simulink model "first_order_system_parabolicC"  (R2022b)
settings: Solver=VariableStepAuto  StartTime=0.0  StopTime=10.0  RelTol=1e-3
settings Model: Creator=yasso  LastModifiedBy=yasso

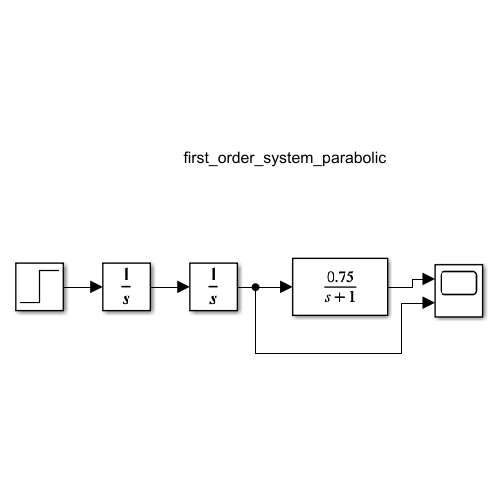
[thumbnail: Simulink's stored preview of the top-level diagram]
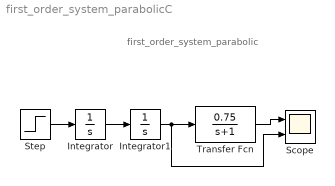
== system first_order_system_parabolicC ==
  note: first_order_system_parabolic
  Integrator : Integrator
  Integrator1 : Integrator
  Scope : Scope  NumInputPorts=2
  Step : Step  SampleTime=0
  Transfer Fcn : TransferFcn  Numerator=[0 0.75]  Denominator=[1 1]
  wires:
  Integrator1/1 -> Scope/2, Transfer Fcn/1
  Integrator/1 -> Integrator1/1
  Step/1 -> Integrator/1
  Transfer Fcn/1 -> Scope/1
